simulink model "test_path_detector"  (Simulink 7.6)
settings: Solver=FixedStepDiscrete  StartTime=0.0  StopTime=0  RelTol=1e-3
values from neighbouring files (symbols this model uses):
  Scale_Down_B = 1    [VisionConstants.m]
  Scale_Down_G = 1    [VisionConstants.m]
  Scale_Down_H = 1    [VisionConstants.m]
  Scale_Down_R = 1    [VisionConstants.m]
  Scale_Down_S = 1    [VisionConstants.m]
  Scale_Down_V = 5    [VisionConstants.m]
undefined symbols (not defined in the file or in its folder): gray, Rec, SDTV
libraries: vipsnks x11, vipconversions x2, viptextngfix x2, vipsrcs x1, viptransforms x1
settings Model: Creator=Thing 1  LastModifiedBy=auvt
settings RTWCC: TargetLang=C++

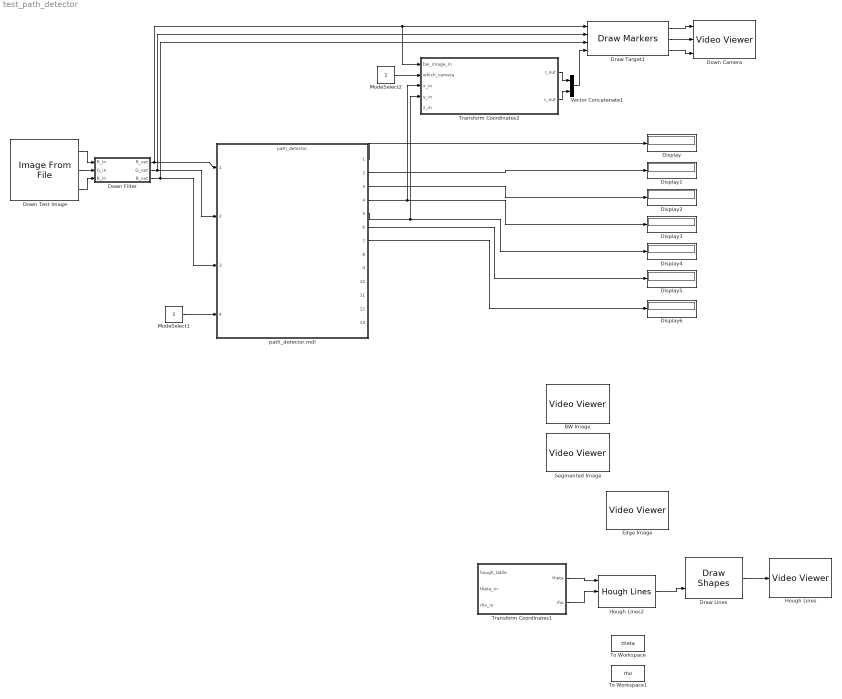
== system test_path_detector ==
  BW Image : vipsnks/Video Viewer  DialogControllerArgs=DataTag1  inputType=Obsolete7b  imagePorts=One multidimensional signal  useColorMap=off  colormapValue=gray(256)  specRange=off  minInputVal=0  maxInputVal=255  FigPos=[632 613 290 272]  AxisZoom=on  trueSizedOnce=off  OpenAtMdlStart=on
  Display{,1..6} (7 alike) : Display
  Down Camera : vipsnks/Video Viewer  DialogControllerArgs=DataTag3  inputType=Obsolete7b  imagePorts=Separate color signals  useColorMap=off  colormapValue=gray(256)  specRange=off  minInputVal=0  maxInputVal=255  FigPos=[733 541 306 217]  AxisZoom=on  trueSizedOnce=off  OpenAtMdlStart=on
  Down Filter : Subsystem
  Down Test Image : vipsrcs/Image From File  Tag=vipblks_nd  DialogController=vipDDGCreate  DialogControllerArgs=DataTag16  SystemSampleTime=-1  FileName=/home/auvt/auvc/src/vision/Test_Images/path9.bmp  imagePorts=Separate color signals  Ts=-1  ImageDataType=double  Signed=on  WordLength=16  sdImageDataType=uint(8)  FractionLengthMode=User-defined  FractionLength=15  OutPortLabels=R|G|B
  Draw Lines : viptextngfix/Draw Shapes  DialogController=vipDDGCreate  DialogControllerArgs=DataTag17  shape=Lines  fill=off  fillClrSource=Specify via dialog  display=User-specified value  intensity=200  color=.5  opacity=0.6  viewport=Entire image  antialiasing=off  inType=Obsolete  imagePorts=One multidimensional signal  prodOutputMode=Binary point scaling  prodOutputWordLength=32  prodOutputFracLength=14  memoryMode=Specify word length  memoryWordLength=16  memoryFracLength=15  roundingMode=Floor  overflowMode=off
  Draw Target1 : viptextngfix/Draw Markers  DialogController=vipDDGCreate  DialogControllerArgs=DataTag18  shape=X-mark  size=7  fill=off  fillClrSource=Specify via dialog  display=User-specified value  intensity=200  color=[0 0 0]  opacity=0.6  viewport=Entire image  antialiasing=off  inType=Obsolete  imagePorts=Separate color signals  prodOutputMode=Binary point scaling  prodOutputWordLength=32  prodOutputFracLength=14  memoryMode=Specify word length  memoryWordLength=16  memoryFracLength=15  roundingMode=Floor  overflowMode=off
  Edge Image : vipsnks/Video Viewer  DialogControllerArgs=DataTag20  inputType=Obsolete7b  imagePorts=One multidimensional signal  useColorMap=off  colormapValue=gray(256)  specRange=off  minInputVal=0  maxInputVal=255  FigPos=[902 374 263 238]  AxisZoom=on  trueSizedOnce=off  OpenAtMdlStart=on
  Hough Lines : vipsnks/Video Viewer  DialogControllerArgs=DataTag22  inputType=Obsolete7b  imagePorts=One multidimensional signal  useColorMap=off  colormapValue=gray(256)  specRange=off  minInputVal=0  maxInputVal=255  FigPos=[698 894 296 325]  AxisZoom=on  trueSizedOnce=off  OpenAtMdlStart=on
  Hough Lines2 : viptransforms/Hough Lines  DialogController=vipDDGCreate  DialogControllerArgs=DataTag23  sineCompMethod=Trigonometric function  thetaRes=pi/180  firstCoeffMode=Specify word length  firstCoeffWordLength=16  firstCoeffFracLength=15  prodOutputMode=Binary point scaling  prodOutputWordLength=32  prodOutputFracLength=16  roundingMode=Nearest  overflowMode=on
  ModeSelect1 : Constant  SampleTime=-1
  ModeSelect2 : Constant  SampleTime=-1
  Segmented Image : vipsnks/Video Viewer  DialogControllerArgs=DataTag25  inputType=Obsolete7b  imagePorts=One multidimensional signal  useColorMap=off  colormapValue=gray(256)  specRange=off  minInputVal=0  maxInputVal=255  FigPos=[964 795 418 649]  AxisZoom=on  trueSizedOnce=off  OpenAtMdlStart=on
  To Workspace : ToWorkspace  VariableName=theta  SampleTime=-1  SaveFormat=Array
  To Workspace1 : ToWorkspace  VariableName=rho  SampleTime=-1  SaveFormat=Array
  Transform Coordinates1 : Stateflow chart  TreatAsAtomicUnit=on  SystemSampleTime=[1/30 0]
  Transform Coordinates2 : Stateflow chart  TreatAsAtomicUnit=on  SystemSampleTime=[1/30 0]
  Vector Concatenate1 : Concatenate  Mode=Multidimensional array
  path_detector.mdl : ModelReference  ModelNameDialog=path_detector  SimulationMode=Accelerator  ModelReferenceVersion=1.223  CopyOfModelName=path_detector
  wires:
  Down Test Image/1 -> Down Filter/1(R_in)
  Down Test Image/2 -> Down Filter/2(G_in)
  Down Test Image/3 -> Down Filter/3(B_in)
  Down Filter/1(R_out) -> Draw Target1/1, Transform Coordinates2/1(bw_image_in), path_detector.mdl/1
  Down Filter/2(G_out) -> Draw Target1/2, path_detector.mdl/2
  Down Filter/3(B_out) -> Draw Target1/3, path_detector.mdl/3
  ModeSelect2/1 -> Transform Coordinates2/2(which_camera)
  Transform Coordinates2/1(r_out) -> Vector Concatenate1/1
  Transform Coordinates2/2(c_out) -> Vector Concatenate1/2
  Vector Concatenate1/1 -> Draw Target1/4
  Draw Target1/1 -> Down Camera/1
  Draw Target1/2 -> Down Camera/2
  Draw Target1/3 -> Down Camera/3
  path_detector.mdl/1 -> Display/1
  path_detector.mdl/2 -> Display1/1
  path_detector.mdl/3 -> Display2/1
  path_detector.mdl/4 -> Display3/1, Transform Coordinates2/3(x_in)
  path_detector.mdl/5 -> Display4/1, Transform Coordinates2/4(y_in)
  path_detector.mdl/6 -> Display5/1
  path_detector.mdl/7 -> Display6/1
  ModeSelect1/1 -> path_detector.mdl/4
  ? -> To Workspace/1
  ? -> To Workspace1/1
  Transform Coordinates1/1(theta) -> Hough Lines2/1
  Transform Coordinates1/2(rho) -> Hough Lines2/2
  Hough Lines2/1 -> Draw Lines/2
  Draw Lines/1 -> Hough Lines/1

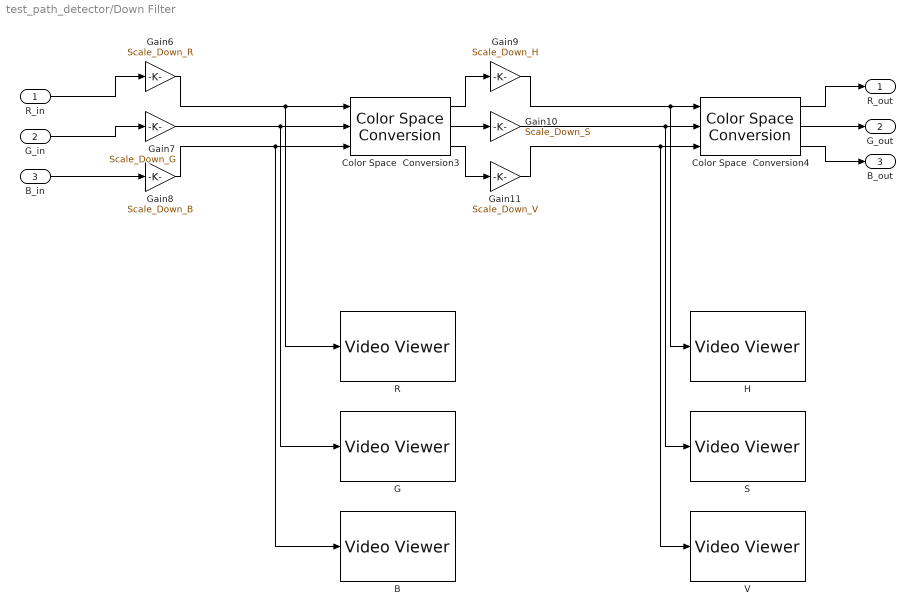
== system test_path_detector/Down Filter ==
  R_in : Inport  PortDimensions=Down_Camera_Dimensions
  G_in : Inport  Port=2  PortDimensions=Down_Camera_Dimensions
  B_in : Inport  Port=3  PortDimensions=Down_Camera_Dimensions
  B : vipsnks/Video Viewer  DialogControllerArgs=DataTag5  inputType=Obsolete7b  imagePorts=One multidimensional signal  useColorMap=off  colormapValue=gray(256)  specRange=off  minInputVal=0  maxInputVal=255  FigPos=[94 842 410 300]  AxisZoom=on  trueSizedOnce=off  OpenAtMdlStart=on
  Color Space  Conversion3 : vipconversions/Color Space  Conversion  conversion=Obsolete  conversionActive=R'G'B' to HSV  wp_str=D50  rec=Rec. 601 (SDTV)  sys=1125/60/2:1  imagePorts=Separate color signals
  Color Space  Conversion4 : vipconversions/Color Space  Conversion  conversion=Obsolete  conversionActive=HSV to R'G'B'  wp_str=D50  rec=Rec. 601 (SDTV)  sys=1125/60/2:1  imagePorts=Separate color signals
  G : vipsnks/Video Viewer  DialogControllerArgs=DataTag7  inputType=Obsolete7b  imagePorts=One multidimensional signal  useColorMap=off  colormapValue=gray(256)  specRange=off  minInputVal=0  maxInputVal=255  FigPos=[111 572 410 300]  AxisZoom=on  trueSizedOnce=off  OpenAtMdlStart=on
  Gain10 : Gain  Gain=Scale_Down_S
  Gain11 : Gain  Gain=Scale_Down_V
  Gain6 : Gain  Gain=Scale_Down_R
  Gain7 : Gain  Gain=Scale_Down_G
  Gain8 : Gain  Gain=Scale_Down_B
  Gain9 : Gain  Gain=Scale_Down_H
  H : vipsnks/Video Viewer  DialogControllerArgs=DataTag9  inputType=Obsolete7b  imagePorts=One multidimensional signal  useColorMap=off  colormapValue=gray(256)  specRange=off  minInputVal=0  maxInputVal=255  FigPos=[439 497 410 300]  AxisZoom=on  trueSizedOnce=off  OpenAtMdlStart=on
  R : vipsnks/Video Viewer  DialogControllerArgs=DataTag11  inputType=Obsolete7b  imagePorts=One multidimensional signal  useColorMap=off  colormapValue=gray(256)  specRange=off  minInputVal=0  maxInputVal=255  FigPos=[30 465 410 300]  AxisZoom=on  trueSizedOnce=off  OpenAtMdlStart=on
  S : vipsnks/Video Viewer  DialogControllerArgs=DataTag13  inputType=Obsolete7b  imagePorts=One multidimensional signal  useColorMap=off  colormapValue=gray(256)  specRange=off  minInputVal=0  maxInputVal=255  FigPos=[475 656 410 300]  AxisZoom=on  trueSizedOnce=off  OpenAtMdlStart=on
  V : vipsnks/Video Viewer  DialogControllerArgs=DataTag15  inputType=Obsolete7b  imagePorts=One multidimensional signal  useColorMap=off  colormapValue=gray(256)  specRange=off  minInputVal=0  maxInputVal=255  FigPos=[504 845 410 300]  AxisZoom=on  trueSizedOnce=off  OpenAtMdlStart=on
  R_out : Outport  OutDataTypeStr=double
  G_out : Outport  Port=2  OutDataTypeStr=double
  B_out : Outport  Port=3  OutDataTypeStr=double
  wires:
  Gain6/1 -> Color Space  Conversion3/1, R/1
  Gain7/1 -> Color Space  Conversion3/2, G/1
  Gain8/1 -> Color Space  Conversion3/3, B/1
  Color Space  Conversion3/1 -> Gain9/1
  Color Space  Conversion3/2 -> Gain10/1
  Color Space  Conversion3/3 -> Gain11/1
  Gain9/1 -> Color Space  Conversion4/1, H/1
  Gain10/1 -> Color Space  Conversion4/2, S/1
  Gain11/1 -> Color Space  Conversion4/3, V/1
  R_in/1 -> Gain6/1
  G_in/1 -> Gain7/1
  B_in/1 -> Gain8/1
  Color Space  Conversion4/1 -> R_out/1
  Color Space  Conversion4/2 -> G_out/1
  Color Space  Conversion4/3 -> B_out/1

== matlab function Transform Coordinates1 ==
  data: hough_table input double; theta_in input double; rho_in input double; theta output double; rho output double
function [theta, rho] = draw_lines(hough_table, theta_in, rho_in)
%#eml

%{
len = min( length(rho_in), length(theta_in) );
rho = zeros(1, len);
theta = zeros(1, len);

for i = 1:len
    rho(i) = rho_in(i);
    theta(i) = theta_in(i);
end
%}



%% Initialize
% Only the (max_num_lines) with the most votes will be considered as
%   candidates for the validation gate
max_num_lines = 50;
[rho_length, theta_length] = size(hough_table);


% These vectors contain intermediate line information; as lines are
%   eliminated from these vectors, their values are set to zero
rho = zeros(1,max_num_lines);
theta = zeros(1,max_num_lines);


% Identify the most popular max_num_lines lines
i_index = ones(1,max_num_lines);
j_index = ones(1,max_num_lines);

m = 1;
while( m <= max_num_lines )
    
    max_votes = 0;
    for i = 1:rho_length
        for j = 1:theta_length
            if( hough_table(i,j) > max_votes )
                i_index(m) = i;
                j_index(m) = j;
                max_votes = hough_table(i,j);
            end
        end
    end
    
    rho(m) = rho_in(i_index(m));
    theta(m) = theta_in(j_index(m));
    hough_table(i_index(m),j_index(m)) = 0;
    m = m + 1;
    
end





return

== matlab function Transform Coordinates2 ==
  data: bw_image_in input double; which_camera input double; x_in input double; y_in input double; r_out output double; c_out output double; z_in input double
function [r_out, c_out] = transform_G2L(bw_image_in, which_camera, x_in, y_in, z_in)
% This function, "transform Global to Local coordinates," transforms
%   global coordinates that are sent to the controller into local
%   coordinates that can be displayed over images.
%
% 5-29-11
%
% Input
%   x_in, y_in, z_in = vectors of points in global (vehicle-centered)
%     coordinate system
%   bw_image_in = a 2-D array of pixel values (used only to extract image
%     size)
%   which_camera = selects which camera for relative coordinates
%                = 0 -> Forward camera
%                = 1 -> Down camera
%
% Output
%   r_out, c_out = row, column pairs in local coordinate system

[rows, cols] = size(bw_image_in);
if( which_camera == 0 )
    r_out = z_in + floor(rows/2);
    c_out = y_in + floor(cols/2);
else
    r_out = floor(rows/2) - x_in;
    c_out = y_in + floor(cols/2);
end

return
